simulink model "Sim_test"  (R2016b)
settings: Solver=ode23tb  StartTime=0.0  StopTime=ti(end)  MaxStep=1e-3  EnableMultiTasking=on
InitFcn:
  | fp_sp_k = 12e3;
  | fp_sp_d = 1;
  | weights = 70/6;
  | joint_k = 0*180/pi;
  | joint_d = 0*180/pi;
  | fp_uj_dp_k = 500*180/pi;
  | fp_uj_dp_d = 1*180/pi;
  | fp_uj_ie_k = 500*180/pi;
  | fp_uj_ie_d = 1*180/pi;
values from neighbouring files (symbols this model uses):
  N = length(shin_angles_in.signals.values)    [GaitEmu_code.m]    (also in dy1.m; dy2.m; est_joint.m = size( [body1.trans body2.trans], 1 ); impcont.m)
  s = [-atan((t2.*3.379e-4+t3+t4.*t5.*4.401e-2)./(t4.*cos(q2)));-asin(t2.*1.4870979e-5+t3.*4.401e-2-t4.*t5)]    [FK_af.m]    (also in FK_footimp.m = [atan((ree2_1.*t2.*4.401e-2+ree2_2.*t4+ree2_3.*t3+t5.*t7.*4.; FK_gaitEmul.m = [q1+t2.*t4.*4.234e-1+t3.*t5.*1.5e-3-t2.*t6.*t7.*1.5e-3-5.347; ik.m = [x; y; z]; ik_af.m = FK_af(q))
  sta = [-0.5345 0.03779 -0.0866]    [GaitEmu_code.m]    (also in dy1.m; dy2.m; grn_dyn.m; impcont.m)
  Y = -( reshape( body1.trans', [], 1 ) - reshape( body2.trans', [], 1 ) )    [creat_joint.m]    (also in est_joint.m = -( reshape( body1.trans', [3*N 1] ) - reshape( body2.trans',)
undefined symbols (not defined in the file or in its folder): X, Z
libraries: sm_lib x263, nesl_utility x76, simulink x3, dspstat3 x1
(part 1 of 6)
settings Model: Creator=lcasteli  LastModifiedBy=Leslie
settings SolverCC: ZeroCrossControl=DisableAll
settings DataIOCC: OutputTimes=[0:0.01:t(end)]
settings OptimizationCC: LifeSpan=inf
settings DebuggingCC: SFUnexpectedBacktrackingDiag=warning  SFNoUnconditionalDefaultTransitionDiag=warning  SFExecutionAtInitializationDiag=none
settings GRTTargetCC: TargetLangStandard=C89/C90 (ANSI)  GeneratePreprocessorConditionals=Disable all
settings ConfigComp: CovMetricSettings=dw  CovHtmlReporting=on  CovSaveCumulativeToWorkspaceVar=on  CovSaveSingleToWorkspaceVar=on  CovExternalEMLEnable=off

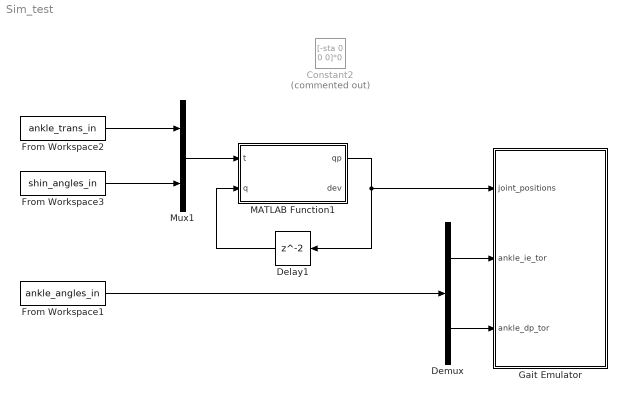
== system Sim_test ==
  Constant2 : Constant  Commented=on  Value=[-sta 0 0 0]*0
  Delay1 : Delay  SampleTime=0.01
  Demux : Demux  Outputs=2
  From Workspace1 : FromWorkspace  VariableName=ankle_angles_in  SampleTime=0
  From Workspace2 : FromWorkspace  VariableName=ankle_trans_in  SampleTime=0
  From Workspace3 : FromWorkspace  VariableName=shin_angles_in  SampleTime=0
  Gait Emulator : Subsystem
  MATLAB Function1 : MATLAB Function  TreatAsAtomicUnit=on
  Mux1 : Mux  Inputs=2
  wires:
  From Workspace1/1 -> Demux/1
  Mux1/1 -> MATLAB Function1/1(t)
  Delay1/1 -> MATLAB Function1/2(q)
  From Workspace2/1 -> Mux1/1
  From Workspace3/1 -> Mux1/2
  MATLAB Function1/1(qp) -> Gait Emulator/1(joint_positions), Delay1/1
  Demux/2 -> Gait Emulator/3(ankle_dp_tor)
  Demux/1 -> Gait Emulator/2(ankle_ie_tor)

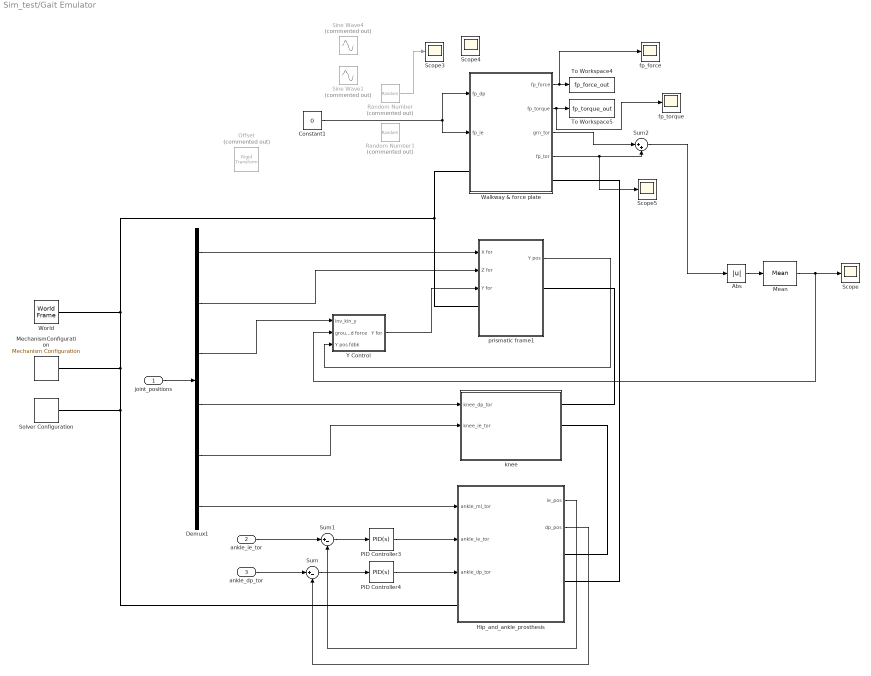
== system Sim_test/Gait Emulator ==
  joint_positions : Inport
  ankle_ie_tor : Inport  Port=2
  ankle_dp_tor : Inport  Port=3
  Abs : Abs
  Constant1 : Constant  Value=0
  Demux1 : Demux  Outputs=6
  Hip_and_ankle_prosthesis : Subsystem
  Mean : dspstat3/Mean  run=off  reset_popup=None  InputProcessing=Columns as channels (frame based)  directionMode=Each column  dimension=1  roiEnable=off  roiType=Rectangles  roiPortion=Entire ROI  roiOutput=Individual statistics for each ROI  roiFlag=off  outputDataTypeStr=Inherit: Same as accumulator  outputLastDataTypeStr=Inherit: Same as accumulator  outputMin=[]  outputMax=[]  roundingMode=Floor  overflowMode=off
  MechanismConfiguration : sm_lib/Utilities/Mechanism Configuration  UniformGravity=Constant  GravityVector=[0 -9.81 0]  GravityUnits=m/s^2  LinearizationDelta=0.001
  Offset : sm_lib/Frames and Transforms/Rigid Transform  Commented=on  TranslationMethod=Cartesian  TranslationStandardOffset=0  TranslationLengthUnit=m  TranslationStandardAxis=+Z  TranslationCartesianOffset=[0.5345 0 -0.03779]  TranslationROffset=0  TranslationROffsetUnits=m  TranslationZOffset=0  TranslationZOffsetUnits=m  TranslationThetaOffset=0  TranslationThetaOffsetUnits=deg  RotationMethod=None  RotationAngleUnits=deg  RotationStandardAxis=+Z  RotationAngle=0.0  RotationArbitraryAxis=[0 0 1]  FollAlignAxisA=+X  BaseAlignAxisA=+Y  FollAlignAxisB=+Y  BaseAlignAxisB=+Z  RotationSequenceAxes=FollowerAxes  RotationSequence=XYX  RotationSequenceAngles=[0 0 0]  RotationSequenceAnglesUnits=deg  RotationMatrix=[1 0 0; 0 1 0; 0 0 1]
  PID Controller3 : simulink/Continuous/PID Controller  Controller=PID  TimeDomain=Continuous-time  SampleTime=-1  IntegratorMethod=Forward Euler  FilterMethod=Forward Euler  Form=Parallel  UseFilter=on  ControllerParametersSource=internal  P=100.231890322584  I=1889.10473464132  D=0.114972413249001  N=105.668461573137  InitialConditionSource=internal  InitialConditionForIntegrator=0  InitialConditionForFilter=0  ExternalReset=none  LimitOutput=off  UpperSaturationLimit=300  LowerSaturationLimit=-300  LinearizeAsGain=on  AntiWindupMode=clamping  Kb=1  TrackingMode=off  Kt=1  PParamMin=[]  PParamMax=[]  IParamMin=[]  IParamMax=[]  DParamMin=[]  DParamMax=[]  NParamMin=[]  NParamMax=[]  KbParamMin=[]  KbParamMax=[]  KtParamMin=[]  KtParamMax=[]  POutMin=[]  POutMax=[]  IOutMin=[]  IOutMax=[]  DOutMin=[]  DOutMax=[]  NOutMin=[]  NOutMax=[]  KbOutMin=[]  KbOutMax=[]  KtOutMin=[]  KtOutMax=[]  IntegratorOutMin=[]  IntegratorOutMax=[]  FilterOutMin=[]  FilterOutMax=[]  SumOutMin=[]  SumOutMax=[]  SumI1OutMin=[]  SumI1OutMax=[]  SumI2OutMin=[]  SumI2OutMax=[]  SumI3OutMin=[]  SumI3OutMax=[]  SumDOutMin=[]  SumDOutMax=[]  SaturationOutMin=[]  SaturationOutMax=[]  IntegratorContinuousStateAttributes=''  IntegratorStateMustResolveToSignalObject=off  IntegratorRTWStateStorageClass=Auto  FilterContinuousStateAttributes=''  FilterStateMustResolveToSignalObject=off  FilterRTWStateStorageClass=Auto  DifferentiatorICPrevScaledInput=0  DifferentiatorOutMin=[]  DifferentiatorOutMax=[]
  PID Controller4 : simulink/Continuous/PID Controller  Controller=PID  TimeDomain=Continuous-time  SampleTime=-1  IntegratorMethod=Forward Euler  FilterMethod=Forward Euler  Form=Parallel  UseFilter=on  ControllerParametersSource=internal  P=98.3049766184944  I=1830.641791322  D=0.171661431514785  N=125.840495387903  InitialConditionSource=internal  InitialConditionForIntegrator=0  InitialConditionForFilter=0  ExternalReset=none  LimitOutput=off  UpperSaturationLimit=300  LowerSaturationLimit=-300  LinearizeAsGain=on  AntiWindupMode=clamping  Kb=1  TrackingMode=off  Kt=1  PParamMin=[]  PParamMax=[]  IParamMin=[]  IParamMax=[]  DParamMin=[]  DParamMax=[]  NParamMin=[]  NParamMax=[]  KbParamMin=[]  KbParamMax=[]  KtParamMin=[]  KtParamMax=[]  POutMin=[]  POutMax=[]  IOutMin=[]  IOutMax=[]  DOutMin=[]  DOutMax=[]  NOutMin=[]  NOutMax=[]  KbOutMin=[]  KbOutMax=[]  KtOutMin=[]  KtOutMax=[]  IntegratorOutMin=[]  IntegratorOutMax=[]  FilterOutMin=[]  FilterOutMax=[]  SumOutMin=[]  SumOutMax=[]  SumI1OutMin=[]  SumI1OutMax=[]  SumI2OutMin=[]  SumI2OutMax=[]  SumI3OutMin=[]  SumI3OutMax=[]  SumDOutMin=[]  SumDOutMax=[]  SaturationOutMin=[]  SaturationOutMax=[]  IntegratorContinuousStateAttributes=''  IntegratorStateMustResolveToSignalObject=off  IntegratorRTWStateStorageClass=Auto  FilterContinuousStateAttributes=''  FilterStateMustResolveToSignalObject=off  FilterRTWStateStorageClass=Auto  DifferentiatorICPrevScaledInput=0  DifferentiatorOutMin=[]  DifferentiatorOutMax=[]
  Random Number : RandomNumber  Commented=on  Variance=1e4  SampleTime=0.1
  Random Number1 : RandomNumber  Commented=on  Variance=4e3  SampleTime=0.1
  Scope{,3..5} (4 alike) : Scope
  Sine Wave1 : Sin  Commented=on  Amplitude=100  Frequency=10  Phase=pi/6  SampleTime=0.001
  Sine Wave4 : Sin  Commented=on  Amplitude=100*2  Frequency=10  SampleTime=0.001
  Solver Configuration : nesl_utility/Solver Configuration  PhysicalDomain=network_engine_domain  SubClassName=solver  LeftPortType=input  RightPortType=generic  Accelerate=off  Tones=[]  Harmonics=[]  SimulateNoise=off  Profile=off  UseLocalSampling=off  EnableSwitchedLinearOptims=on  FrequencyDomain=off  UseCCode=off  RelTol=0.001  AbsTol=1e-06  MinStep=1e-09  ToWorkspace=off  RevertToSquareIcSolve=off  NumHomotopyIterations=100  PhasorMode=off  PhasorModeNumHarmonics=1  OverrideAbsTol=off  DoDC=off  ResidualTolerance=1e-09  UseLocalSolver=off  LocalSolverChoice=NE_BACKWARD_EULER_ADVANCER  LocalSolverSampleTime=0.001  DoFixedCost=off  MaxNonlinIter=3  MaxModeIter=2  LinearAlgebra=Sparse  DelaysMemoryBudget=1024  AutomaticFiltering=on  FilteringTimeConstant=0.001
  Sum : Sum  Inputs=|+-
  Sum1 : Sum  Inputs=|+-
  Sum2 : Sum  Inputs=|++
  To Workspace4 : ToWorkspace  VariableName=fp_force_out  SaveFormat=Structure With Time  SampleTime=-1
  To Workspace5 : ToWorkspace  VariableName=fp_torque_out  SaveFormat=Structure With Time  SampleTime=-1
  Walkway & force plate : Subsystem
  World : sm_lib/Frames and Transforms/World Frame
  Y Control : Subsystem
  fp_force : Scope
  fp_torque : Scope
  "knee " : Subsystem
  prismatic frame1 : Subsystem
  wires:
  joint_positions/1 -> Demux1/1
  Walkway & force plate/2(fp_torque) -> fp_torque/1, To Workspace5/1
  Walkway & force plate/1(fp_force) -> fp_force/1, To Workspace4/1
  Demux1/4 -> "knee "/1(knee_dp_tor)
  Demux1/5 -> "knee "/2(knee_ie_tor)
  Demux1/6 -> Hip_and_ankle_prosthesis/1(ankle_ml_tor)
  Walkway & force plate/3(grn_tor) -> Sum2/1
  Walkway & force plate/4(fp_tor) -> Scope5/1, Sum2/2
  Sum2/1 -> Abs/1
  Abs/1 -> Mean/1
  Mean/1 -> Y Control/2(ground force), Scope/1
  Hip_and_ankle_prosthesis/2(dp_pos) -> Sum/2
  Hip_and_ankle_prosthesis/1(ie_pos) -> Sum1/2
  Sum1/1 -> PID Controller3/1
  Sum/1 -> PID Controller4/1
  Random Number/1 -> Scope3/1
  Constant1/1 -> Walkway & force plate/2(fp_ie), Walkway & force plate/1(fp_dp)
  prismatic frame1/1(Y pos) -> Y Control/3(Y pos fdbk)
  Y Control/1(Y for) -> prismatic frame1/3(Y for)
  Demux1/1 -> prismatic frame1/1(X for)
  Demux1/2 -> prismatic frame1/2(Z for)
  Demux1/3 -> Y Control/1(inv_kin_y)
  PID Controller3/1 -> Hip_and_ankle_prosthesis/2(ankle_ie_tor)
  PID Controller4/1 -> Hip_and_ankle_prosthesis/3(ankle_dp_tor)
  ankle_dp_tor/1 -> Sum/1
  ankle_ie_tor/1 -> Sum1/1
  connections:
  Hip_and_ankle_prosthesis/RConn1 -- "knee "/RConn2
  Walkway & force plate/RConn1 -- Hip_and_ankle_prosthesis/RConn2
  Walkway & force plate/LConn1 -- prismatic frame1/LConn1 -- Hip_and_ankle_prosthesis/LConn1 -- Solver Configuration/RConn1 -- MechanismConfiguration/RConn1 -- World/RConn1
  prismatic frame1/RConn1 -- "knee "/RConn1

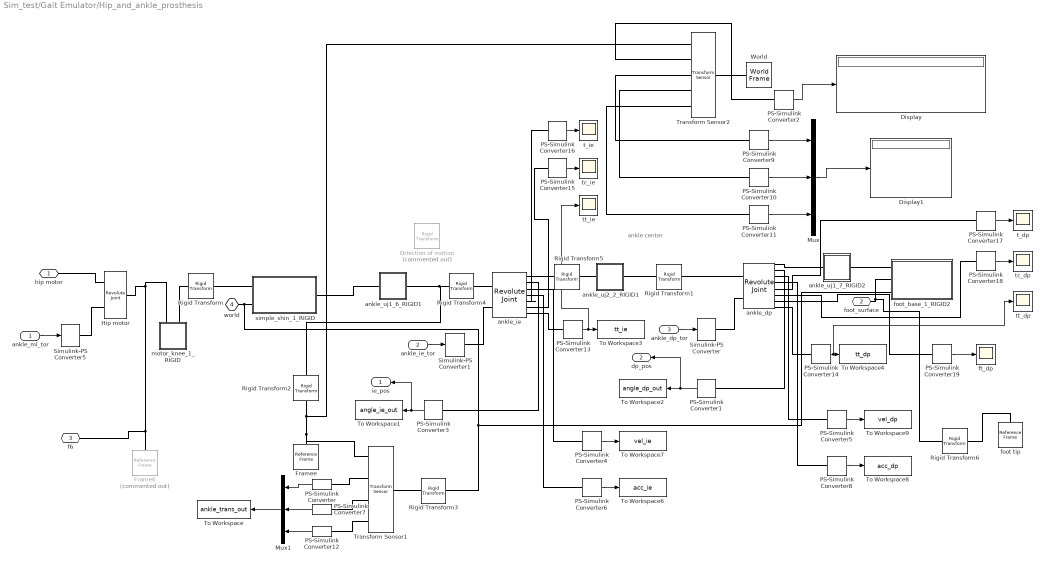
== system Sim_test/Gait Emulator/Hip_and_ankle_prosthesis ==
  note: ankle center
  ankle_ml_tor : Inport
  ankle_ie_tor : Inport  Port=2
  ankle_dp_tor : Inport  Port=3
  Display : Display
  Display1 : Display
  Driection of motion : sm_lib/Frames and Transforms/Rigid Transform  Commented=on  TranslationMethod=None  TranslationStandardOffset=0  TranslationLengthUnit=m  TranslationStandardAxis=+Z  TranslationCartesianOffset=[0 0 0]  TranslationROffset=0  TranslationROffsetUnits=m  TranslationZOffset=0  TranslationZOffsetUnits=m  TranslationThetaOffset=0  TranslationThetaOffsetUnits=deg  RotationMethod=StandardAxis  RotationAngleUnits=deg  RotationStandardAxis=+Z  RotationAngle=0  RotationArbitraryAxis=[0 0 1]  FollAlignAxisA=+X  BaseAlignAxisA=+Y  FollAlignAxisB=+Y  BaseAlignAxisB=+Z  RotationSequenceAxes=FollowerAxes  RotationSequence=XYX  RotationSequenceAngles=[0 0 0]  RotationSequenceAnglesUnits=deg  RotationMatrix=[1 0 0; 0 1 0; 0 0 1]
  Frame6 : sm_lib/Frames and Transforms/Reference Frame  Commented=on
  Framee : sm_lib/Frames and Transforms/Reference Frame
  Hip motor : sm_lib/Joints/Revolute Joint  SenseConstraintForce=off  SenseConstraintForceX=off  SenseConstraintForceY=off  SenseConstraintForceZ=off  SenseConstraintTorque=off  SenseConstraintTorqueX=off  SenseConstraintTorqueY=off  SenseConstraintTorqueZ=off  SenseTotalForce=off  SenseTotalForceX=off  SenseTotalForceY=off  SenseTotalForceZ=off  SenseTotalTorque=off  SenseTotalTorqueX=off  SenseTotalTorqueY=off  SenseTotalTorqueZ=off  CompositeWrenchDir=FollowerOnBase  CompositeWrenchFrame=BaseFrame  EquilibriumPosition=0  EquilibriumPositionUnits=rad  SpringStiffness=joint_k  SpringStiffnessUnits=m*N/rad  DampingCoefficient=joint_d  DampingCoefficientUnits=m*s*N/rad  TorqueActuationMode=ComputedTorque  MotionActuationMode=InputMotion  SensePosition=off  SenseVelocity=off  SenseAcceleration=off  SenseTorqueForce=off  PositionTargetSpecify=off  PositionTargetPriority=Low  PositionTargetValue=0  PositionTargetValueUnits=deg  VelocityTargetSpecify=off  VelocityTargetPriority=High  VelocityTargetValue=0  VelocityTargetValueUnits=deg/s
  Mux : Mux  Inputs=3
  Mux1 : Mux  Inputs=3
  PS-Simulink Converter{,1..19} (20 alike) : nesl_utility/PS-Simulink Converter  PhysicalDomain=network_engine_domain  SubClassName=ps_output  LeftPortType=input  RightPortType=output  PseudoPeriodic=off  Frequencies=[]  Unit=1  AffineConversion=off
  Rigid Transform : sm_lib/Frames and Transforms/Rigid Transform  TranslationMethod=StandardAxis  TranslationStandardOffset=0.15  TranslationLengthUnit=m  TranslationStandardAxis=+Z  TranslationCartesianOffset=[0 0 0]  TranslationROffset=0  TranslationROffsetUnits=m  TranslationZOffset=0  TranslationZOffsetUnits=m  TranslationThetaOffset=0  TranslationThetaOffsetUnits=deg  RotationMethod=StandardAxis  RotationAngleUnits=deg  RotationStandardAxis=+X  RotationAngle=180  RotationArbitraryAxis=[1 0 1]  FollAlignAxisA=+X  BaseAlignAxisA=+Y  FollAlignAxisB=+Y  BaseAlignAxisB=+Z  RotationSequenceAxes=FollowerAxes  RotationSequence=XYX  RotationSequenceAngles=[0 0 0]  RotationSequenceAnglesUnits=deg  RotationMatrix=[1 0 0; 0 1 0; 0 0 1]
  Rigid Transform1 : sm_lib/Frames and Transforms/Rigid Transform  TranslationMethod=None  TranslationStandardOffset=0.15  TranslationLengthUnit=m  TranslationStandardAxis=+Z  TranslationCartesianOffset=[0 0 0]  TranslationROffset=0  TranslationROffsetUnits=m  TranslationZOffset=0  TranslationZOffsetUnits=m  TranslationThetaOffset=0  TranslationThetaOffsetUnits=deg  RotationMethod=StandardAxis  RotationAngleUnits=deg  RotationStandardAxis=+Z  RotationAngle=-90  RotationArbitraryAxis=[1 0 1]  FollAlignAxisA=+X  BaseAlignAxisA=+Y  FollAlignAxisB=+Y  BaseAlignAxisB=+Z  RotationSequenceAxes=FollowerAxes  RotationSequence=XYX  RotationSequenceAngles=[0 0 0]  RotationSequenceAnglesUnits=deg  RotationMatrix=[1 0 0; 0 1 0; 0 0 1]
  Rigid Transform2 : sm_lib/Frames and Transforms/Rigid Transform  TranslationMethod=StandardAxis  TranslationStandardOffset=-8.5e-3  TranslationLengthUnit=m  TranslationStandardAxis=+Z  TranslationCartesianOffset=[0 0 0]  TranslationROffset=0  TranslationROffsetUnits=m  TranslationZOffset=0  TranslationZOffsetUnits=m  TranslationThetaOffset=0  TranslationThetaOffsetUnits=deg  RotationMethod=AlignedAxes  RotationAngleUnits=deg  RotationStandardAxis=+Z  RotationAngle=-90  RotationArbitraryAxis=[1 0 1]  FollAlignAxisA=+X  BaseAlignAxisA=-Z  FollAlignAxisB=+Y  BaseAlignAxisB=-Y  RotationSequenceAxes=FollowerAxes  RotationSequence=XYX  RotationSequenceAngles=[0 0 0]  RotationSequenceAnglesUnits=deg  RotationMatrix=[1 0 0; 0 1 0; 0 0 1]
  Rigid Transform3 : sm_lib/Frames and Transforms/Rigid Transform  TranslationMethod=StandardAxis  TranslationStandardOffset=0.1517  TranslationLengthUnit=m  TranslationStandardAxis=+Y  TranslationCartesianOffset=[0 0 0]  TranslationROffset=0  TranslationROffsetUnits=m  TranslationZOffset=0  TranslationZOffsetUnits=m  TranslationThetaOffset=0  TranslationThetaOffsetUnits=deg  RotationMethod=None  RotationAngleUnits=deg  RotationStandardAxis=+Z  RotationAngle=0.0  RotationArbitraryAxis=[0 0 1]  FollAlignAxisA=+X  BaseAlignAxisA=+Y  FollAlignAxisB=+Y  BaseAlignAxisB=+Z  RotationSequenceAxes=FollowerAxes  RotationSequence=XYX  RotationSequenceAngles=[0 0 0]  RotationSequenceAnglesUnits=deg  RotationMatrix=[1 0 0; 0 1 0; 0 0 1]
  Rigid Transform4 : sm_lib/Frames and Transforms/Rigid Transform  TranslationMethod=StandardAxis  TranslationStandardOffset=-8.5e-3  TranslationLengthUnit=m  TranslationStandardAxis=+Z  TranslationCartesianOffset=[0 0 0]  TranslationROffset=0  TranslationROffsetUnits=m  TranslationZOffset=0  TranslationZOffsetUnits=m  TranslationThetaOffset=0  TranslationThetaOffsetUnits=deg  RotationMethod=None  RotationAngleUnits=deg  RotationStandardAxis=+Z  RotationAngle=0.0  RotationArbitraryAxis=[0 0 1]  FollAlignAxisA=+X  BaseAlignAxisA=+Y  FollAlignAxisB=+Y  BaseAlignAxisB=+Z  RotationSequenceAxes=FollowerAxes  RotationSequence=XYX  RotationSequenceAngles=[0 0 0]  RotationSequenceAnglesUnits=deg  RotationMatrix=[1 0 0; 0 1 0; 0 0 1]
  Rigid Transform5 : sm_lib/Frames and Transforms/Rigid Transform  TranslationMethod=StandardAxis  TranslationStandardOffset=8.5e-3  TranslationLengthUnit=m  TranslationStandardAxis=+Z  TranslationCartesianOffset=[0 0 0]  TranslationROffset=0  TranslationROffsetUnits=m  TranslationZOffset=0  TranslationZOffsetUnits=m  TranslationThetaOffset=0  TranslationThetaOffsetUnits=deg  RotationMethod=None  RotationAngleUnits=deg  RotationStandardAxis=+Z  RotationAngle=0.0  RotationArbitraryAxis=[0 0 1]  FollAlignAxisA=+X  BaseAlignAxisA=+Y  FollAlignAxisB=+Y  BaseAlignAxisB=+Z  RotationSequenceAxes=FollowerAxes  RotationSequence=XYX  RotationSequenceAngles=[0 0 0]  RotationSequenceAnglesUnits=deg  RotationMatrix=[1 0 0; 0 1 0; 0 0 1]
  Rigid Transform6 : sm_lib/Frames and Transforms/Rigid Transform  TranslationMethod=StandardAxis  TranslationStandardOffset=-0.181  TranslationLengthUnit=m  TranslationStandardAxis=+X  TranslationCartesianOffset=[0 0 0]  TranslationROffset=0  TranslationROffsetUnits=m  TranslationZOffset=0  TranslationZOffsetUnits=m  TranslationThetaOffset=0  TranslationThetaOffsetUnits=deg  RotationMethod=None  RotationAngleUnits=deg  RotationStandardAxis=+Z  RotationAngle=0.0  RotationArbitraryAxis=[0 0 1]  FollAlignAxisA=+X  BaseAlignAxisA=+Y  FollAlignAxisB=+Y  BaseAlignAxisB=+Z  RotationSequenceAxes=FollowerAxes  RotationSequence=XYX  RotationSequenceAngles=[0 0 0]  RotationSequenceAnglesUnits=deg  RotationMatrix=[1 0 0; 0 1 0; 0 0 1]
  Simulink-PS Converter : nesl_utility/Simulink-PS Converter  PhysicalDomain=network_engine_domain  SubClassName=ps_input  LeftPortType=input  RightPortType=output  PseudoPeriodic=off  Frequencies=[]  NoiseDistribution=none  NoiseParameters=[]  Unit=1  AffineConversion=off  InputFiltering=on  SimscapeFilterOrder=2  InputFilterTimeConstant=0.001  UdotUserProvided=1
  Simulink-PS Converter1 : nesl_utility/Simulink-PS Converter  PhysicalDomain=network_engine_domain  SubClassName=ps_input  LeftPortType=input  RightPortType=output  PseudoPeriodic=off  Frequencies=[]  NoiseDistribution=none  NoiseParameters=[]  Unit=1  AffineConversion=off  InputFiltering=on  SimscapeFilterOrder=2  InputFilterTimeConstant=0.001  UdotUserProvided=2
  Simulink-PS Converter5 : nesl_utility/Simulink-PS Converter  PhysicalDomain=network_engine_domain  SubClassName=ps_input  LeftPortType=input  RightPortType=output  PseudoPeriodic=off  Frequencies=[]  NoiseDistribution=none  NoiseParameters=[]  Unit=1  AffineConversion=off  InputFiltering=on  SimscapeFilterOrder=2  InputFilterTimeConstant=0.001  UdotUserProvided=2
  To Workspace : ToWorkspace  VariableName=ankle_trans_out  SaveFormat=Structure With Time  SampleTime=-1
  To Workspace1 : ToWorkspace  VariableName=angle_ie_out  SaveFormat=Structure With Time  SampleTime=-1
  To Workspace2 : ToWorkspace  VariableName=angle_dp_out  SaveFormat=Structure With Time  SampleTime=-1
  To Workspace3 : ToWorkspace  VariableName=tt_ie  SaveFormat=Structure With Time  SampleTime=-1
  To Workspace4 : ToWorkspace  VariableName=tt_dp  SaveFormat=Structure With Time  SampleTime=-1
  To Workspace6 : ToWorkspace  VariableName=acc_ie  SaveFormat=Structure With Time  SampleTime=-1
  To Workspace7 : ToWorkspace  VariableName=vel_ie  SaveFormat=Structure With Time  SampleTime=-1
  To Workspace8 : ToWorkspace  VariableName=acc_dp  SaveFormat=Structure With Time  SampleTime=-1
  To Workspace9 : ToWorkspace  VariableName=vel_dp  SaveFormat=Structure With Time  SampleTime=-1
  Transform Sensor1 : sm_lib/Frames and Transforms/Transform Sensor  MeasurementFrame=Base  SenseAngle=off  SenseAxis=off  SenseAngle1=off  SenseAngle2=off  SenseAngle3=off  SenseQ=off  SenseR=off  SenseOmegaX=off  SenseOmegaY=off  SenseOmegaZ=off  SenseOmega1=off  SenseOmega2=off  SenseOmega3=off  SenseQDot=off  SenseRDot=off  SenseAlphaX=off  SenseAlphaY=off  SenseAlphaZ=off  SenseAlpha1=off  SenseAlpha2=off  SenseAlpha3=off  SenseQDDot=off  SenseRDDot=off  SenseX=on  SenseY=on  SenseZ=on  SenseRad=off  SenseAzim=off  SenseDist=off  SenseInc=off  SenseXDot=off  SenseYDot=off  SenseZDot=off  SenseRadDot=off  SenseAzimDot=off  SenseDistDot=off  SenseIncDot=off  SenseXDDot=off  SenseYDDot=off  SenseZDDot=off  SenseRadDDot=off  SenseAzimDDot=off  SenseDistDDot=off  SenseIncDDot=off
  Transform Sensor2 : sm_lib/Frames and Transforms/Transform Sensor  MeasurementFrame=Base  SenseAngle=off  SenseAxis=off  SenseAngle1=off  SenseAngle2=off  SenseAngle3=off  SenseQ=off  SenseR=on  SenseOmegaX=off  SenseOmegaY=off  SenseOmegaZ=off  SenseOmega1=off  SenseOmega2=off  SenseOmega3=off  SenseQDot=off  SenseRDot=off  SenseAlphaX=off  SenseAlphaY=off  SenseAlphaZ=off  SenseAlpha1=off  SenseAlpha2=off  SenseAlpha3=off  SenseQDDot=off  SenseRDDot=off  SenseX=on  SenseY=on  SenseZ=on  SenseRad=off  SenseAzim=off  SenseDist=off  SenseInc=off  SenseXDot=off  SenseYDot=off  SenseZDot=off  SenseRadDot=off  SenseAzimDot=off  SenseDistDot=off  SenseIncDot=off  SenseXDDot=off  SenseYDDot=off  SenseZDDot=off  SenseRadDDot=off  SenseAzimDDot=off  SenseDistDDot=off  SenseIncDDot=off
  World : sm_lib/Frames and Transforms/World Frame
  ankle_dp : sm_lib/Joints/Revolute Joint  SenseConstraintForce=off  SenseConstraintForceX=off  SenseConstraintForceY=off  SenseConstraintForceZ=off  SenseConstraintTorque=on  SenseConstraintTorqueX=off  SenseConstraintTorqueY=off  SenseConstraintTorqueZ=off  SenseTotalForce=on  SenseTotalForceX=off  SenseTotalForceY=off  SenseTotalForceZ=off  SenseTotalTorque=on  SenseTotalTorqueX=off  SenseTotalTorqueY=off  SenseTotalTorqueZ=off  CompositeWrenchDir=FollowerOnBase  CompositeWrenchFrame=BaseFrame  EquilibriumPosition=0  EquilibriumPositionUnits=rad  SpringStiffness=stiff_dp  SpringStiffnessUnits=m*N/rad  DampingCoefficient=damp_dp  DampingCoefficientUnits=m*s*N/rad  TorqueActuationMode=InputTorque  MotionActuationMode=ComputedMotion  SensePosition=on  SenseVelocity=on  SenseAcceleration=on  SenseTorqueForce=on  PositionTargetSpecify=off  PositionTargetPriority=Low  PositionTargetValue=-90  PositionTargetValueUnits=deg  VelocityTargetSpecify=off  VelocityTargetPriority=High  VelocityTargetValue=0  VelocityTargetValueUnits=deg/s
  ankle_ie : sm_lib/Joints/Revolute Joint  SenseConstraintForce=off  SenseConstraintForceX=off  SenseConstraintForceY=off  SenseConstraintForceZ=off  SenseConstraintTorque=on  SenseConstraintTorqueX=off  SenseConstraintTorqueY=off  SenseConstraintTorqueZ=off  SenseTotalForce=off  SenseTotalForceX=off  SenseTotalForceY=off  SenseTotalForceZ=off  SenseTotalTorque=on  SenseTotalTorqueX=off  SenseTotalTorqueY=off  SenseTotalTorqueZ=off  CompositeWrenchDir=FollowerOnBase  CompositeWrenchFrame=BaseFrame  EquilibriumPosition=0  EquilibriumPositionUnits=rad  SpringStiffness=stiff_ie  SpringStiffnessUnits=N*m/rad  DampingCoefficient=damp_ie  DampingCoefficientUnits=m*s*N/rad  TorqueActuationMode=InputTorque  MotionActuationMode=ComputedMotion  SensePosition=on  SenseVelocity=on  SenseAcceleration=on  SenseTorqueForce=on  PositionTargetSpecify=off  PositionTargetPriority=Low  PositionTargetValue=0  PositionTargetValueUnits=deg  VelocityTargetSpecify=off  VelocityTargetPriority=High  VelocityTargetValue=0  VelocityTargetValueUnits=deg/s
  ankle_uj1_6_RIGID1 : Subsystem
  ankle_uj1_7_RIGID2 : Subsystem
  ankle_uj2_2_RIGID1 : Subsystem
  foot tip : sm_lib/Frames and Transforms/Reference Frame
  foot_base_1_RIGID2 : Subsystem
  ft_dp : Scope
  motor_knee_1_RIGID : Subsystem
  simple_shin_1_RIGID : Subsystem
  t_dp : Scope
  t_ie : Scope
  tc_dp : Scope
  tc_ie : Scope
  tt_dp : Scope
  tt_ie : Scope
  hip motor : PMIOPort  Port=1  Side=Right
  foot_surface : PMIOPort  Port=2  Side=Right
  f6 : PMIOPort  Port=3  Side=Right
  world : PMIOPort  Port=4  Side=Left
  ie_pos : Outport
  dp_pos : Outport  Port=2
  wires:
  PS-Simulink Converter1/1 -> dp_pos/1, To Workspace2/1
  PS-Simulink Converter4/1 -> To Workspace7/1
  PS-Simulink Converter5/1 -> To Workspace9/1
  PS-Simulink Converter6/1 -> To Workspace6/1
  PS-Simulink Converter8/1 -> To Workspace8/1
  PS-Simulink Converter9/1 -> Mux/1
  PS-Simulink Converter10/1 -> Mux/2
  PS-Simulink Converter11/1 -> Mux/3
  Mux/1 -> Display1/1
  ankle_ml_tor/1 -> Simulink-PS Converter5/1
  PS-Simulink Converter2/1 -> Display/1
  PS-Simulink Converter3/1 -> ie_pos/1, To Workspace1/1
  ankle_dp_tor/1 -> Simulink-PS Converter/1
  PS-Simulink Converter/1 -> Mux1/1
  PS-Simulink Converter7/1 -> Mux1/2
  PS-Simulink Converter12/1 -> Mux1/3
  Mux1/1 -> To Workspace/1
  PS-Simulink Converter13/1 -> tt_ie/1, To Workspace3/1
  PS-Simulink Converter14/1 -> tt_dp/1, To Workspace4/1
  PS-Simulink Converter18/1 -> tc_dp/1
  PS-Simulink Converter17/1 -> t_dp/1
  PS-Simulink Converter15/1 -> tc_ie/1
  PS-Simulink Converter16/1 -> t_ie/1
  ankle_ie_tor/1 -> Simulink-PS Converter1/1
  PS-Simulink Converter19/1 -> ft_dp/1
  connections:
  ankle_uj2_2_RIGID1/LConn1 -- Rigid Transform5/RConn1
  Rigid Transform1/RConn1 -- ankle_dp/LConn1
  simple_shin_1_RIGID/LConn1 -- Rigid Transform/RConn1
  Rigid Transform/LConn1 -- motor_knee_1_RIGID/RConn2
  ankle_uj2_2_RIGID1/RConn1 -- Rigid Transform1/LConn1
  Hip motor/RConn1 -- motor_knee_1_RIGID/RConn1 -- Frame6/RConn1 -- f6/RConn1
  Hip motor/LConn1 -- hip motor/RConn1
  PS-Simulink Converter4/LConn1 -- ankle_ie/RConn3
  PS-Simulink Converter5/LConn1 -- ankle_dp/RConn3
  PS-Simulink Converter6/LConn1 -- ankle_ie/RConn4
  PS-Simulink Converter8/LConn1 -- ankle_dp/RConn4
  foot_base_1_RIGID2/LConn1 -- ankle_uj1_7_RIGID2/RConn1
  ankle_uj1_7_RIGID2/LConn1 -- ankle_dp/RConn1
  foot_base_1_RIGID2/LConn2 -- Rigid Transform6/LConn1 -- foot_surface/RConn1
  PS-Simulink Converter3/LConn1 -- ankle_ie/RConn2
  PS-Simulink Converter1/LConn1 -- ankle_dp/RConn2
  Transform Sensor2/LConn1 -- World/RConn1
  Transform Sensor2/RConn2 -- PS-Simulink Converter2/LConn1
  Transform Sensor2/RConn3 -- PS-Simulink Converter9/LConn1
  Transform Sensor2/RConn4 -- PS-Simulink Converter10/LConn1
  Transform Sensor2/RConn5 -- PS-Simulink Converter11/LConn1
  Framee/RConn1 -- Rigid Transform2/RConn1 -- Transform Sensor2/RConn1 -- Transform Sensor1/RConn1
  simple_shin_1_RIGID/RConn1 -- ankle_uj1_6_RIGID1/LConn1
  Rigid Transform3/RConn1 -- Transform Sensor1/LConn1
  Transform Sensor1/RConn2 -- PS-Simulink Converter/LConn1
  Transform Sensor1/RConn3 -- PS-Simulink Converter7/LConn1
  Transform Sensor1/RConn4 -- PS-Simulink Converter12/LConn1
  ankle_ie/RConn6 -- PS-Simulink Converter15/LConn1
  ankle_ie/RConn7 -- PS-Simulink Converter13/LConn1
  ankle_ie/RConn5 -- PS-Simulink Converter16/LConn1
  ankle_dp/RConn5 -- PS-Simulink Converter17/LConn1
  ankle_dp/RConn6 -- PS-Simulink Converter18/LConn1
  Rigid Transform2/LConn1 -- ankle_uj1_6_RIGID1/RConn1 -- Rigid Transform4/LConn1
  Rigid Transform4/RConn1 -- ankle_ie/LConn1
  Rigid Transform5/LConn1 -- ankle_ie/RConn1
  ankle_dp/LConn2 -- Simulink-PS Converter/RConn1
  world/RConn1 -- Rigid Transform3/LConn1 -- foot_base_1_RIGID2/LConn3 -- simple_shin_1_RIGID/LConn2
  Simulink-PS Converter5/RConn1 -- Hip motor/LConn2
  ankle_ie/LConn2 -- Simulink-PS Converter1/RConn1
  PS-Simulink Converter14/LConn1 -- ankle_dp/RConn8
  PS-Simulink Converter19/LConn1 -- ankle_dp/RConn7
  Rigid Transform6/RConn1 -- foot tip/RConn1

== system Sim_test/Gait Emulator/Walkway & force plate ==
  fp_dp : Inport
  fp_ie : Inport  Port=2
  FP Contact : Subsystem
  Force Plate : Subsystem
  Ground Contact : Subsystem
  Simulink-PS Converter3 : nesl_utility/Simulink-PS Converter  PhysicalDomain=network_engine_domain  SubClassName=ps_input  LeftPortType=input  RightPortType=output  PseudoPeriodic=off  Frequencies=[]  NoiseDistribution=none  NoiseParameters=[]  Unit=1  AffineConversion=off  InputFiltering=on  SimscapeFilterOrder=2  InputFilterTimeConstant=0.001  UdotUserProvided=1
  Simulink-PS Converter7 : nesl_utility/Simulink-PS Converter  PhysicalDomain=network_engine_domain  SubClassName=ps_input  LeftPortType=input  RightPortType=output  PseudoPeriodic=off  Frequencies=[]  NoiseDistribution=none  NoiseParameters=[]  Unit=1  AffineConversion=off  InputFiltering=on  SimscapeFilterOrder=2  InputFilterTimeConstant=0.0001  UdotUserProvided=1
  Transform2 : sm_lib/Frames and Transforms/Rigid Transform  TranslationMethod=StandardAxis  TranslationStandardOffset=0.1517  TranslationLengthUnit=m  TranslationStandardAxis=+Y  TranslationCartesianOffset=[0 0 0]  TranslationROffset=0  TranslationROffsetUnits=m  TranslationZOffset=0  TranslationZOffsetUnits=m  TranslationThetaOffset=0  TranslationThetaOffsetUnits=deg  RotationMethod=StandardAxis  RotationAngleUnits=deg  RotationStandardAxis=+X  RotationAngle=-90  RotationArbitraryAxis=[0 0 1]  FollAlignAxisA=+X  BaseAlignAxisA=+Y  FollAlignAxisB=+Y  BaseAlignAxisB=+Z  RotationSequenceAxes=FollowerAxes  RotationSequence=XYX  RotationSequenceAngles=[0 0 0]  RotationSequenceAnglesUnits=deg  RotationMatrix=[1 0 0; 0 1 0; 0 0 1]
  walkway_1_RIGID : Subsystem
  world : PMIOPort  Port=1  Side=Left
  foot surface : PMIOPort  Port=2  Side=Right
  fp_force : Outport
  fp_torque : Outport  Port=2
  grn_tor : Outport  Port=3
  fp_tor : Outport  Port=4
  wires:
  fp_dp/1 -> Simulink-PS Converter3/1
  fp_ie/1 -> Simulink-PS Converter7/1
  Force Plate/1(fp_force) -> fp_force/1
  Force Plate/2(fp_torque) -> fp_torque/1
  Ground Contact/1(grn_tor) -> grn_tor/1
  FP Contact/1(fp_tor) -> fp_tor/1
  connections:
  Force Plate/RConn1 -- FP Contact/RConn1
  FP Contact/LConn1 -- Ground Contact/LConn1 -- foot surface/RConn1
  Ground Contact/RConn1 -- Transform2/RConn1
  Simulink-PS Converter3/RConn1 -- Force Plate/LConn2
  Force Plate/LConn3 -- Simulink-PS Converter7/RConn1
  Transform2/LConn1 -- walkway_1_RIGID/LConn1 -- Force Plate/LConn1 -- world/RConn1

== system Sim_test/Gait Emulator/Y Control ==
  inv_kin_y : Inport
  ground force : Inport  Port=2
  Y pos fdbk : Inport  Port=3
  Constant : Constant  Value=0
  PID Controller2 : simulink/Continuous/PID Controller  Controller=PID  TimeDomain=Continuous-time  SampleTime=-1  IntegratorMethod=Forward Euler  FilterMethod=Forward Euler  Form=Parallel  UseFilter=on  ControllerParametersSource=internal  P=81311.420853362  I=160476.881141818  D=5207.81218139461  N=8271.05073782612  InitialConditionSource=internal  InitialConditionForIntegrator=0  InitialConditionForFilter=0  ExternalReset=none  LimitOutput=on  UpperSaturationLimit=2*75*9.81  LowerSaturationLimit=-2*75*9.81  LinearizeAsGain=on  AntiWindupMode=clamping  Kb=1  TrackingMode=off  Kt=1  PParamMin=[]  PParamMax=[]  IParamMin=[]  IParamMax=[]  DParamMin=[]  DParamMax=[]  NParamMin=[]  NParamMax=[]  KbParamMin=[]  KbParamMax=[]  KtParamMin=[]  KtParamMax=[]  POutMin=[]  POutMax=[]  IOutMin=[]  IOutMax=[]  DOutMin=[]  DOutMax=[]  NOutMin=[]  NOutMax=[]  KbOutMin=[]  KbOutMax=[]  KtOutMin=[]  KtOutMax=[]  IntegratorOutMin=[]  IntegratorOutMax=[]  FilterOutMin=[]  FilterOutMax=[]  SumOutMin=[]  SumOutMax=[]  SumI1OutMin=[]  SumI1OutMax=[]  SumI2OutMin=[]  SumI2OutMax=[]  SumI3OutMin=[]  SumI3OutMax=[]  SumDOutMin=[]  SumDOutMax=[]  SaturationOutMin=[]  SaturationOutMax=[]  IntegratorContinuousStateAttributes=''  IntegratorStateMustResolveToSignalObject=off  IntegratorRTWStateStorageClass=Auto  FilterContinuousStateAttributes=''  FilterStateMustResolveToSignalObject=off  FilterRTWStateStorageClass=Auto  DifferentiatorICPrevScaledInput=0  DifferentiatorOutMin=[]  DifferentiatorOutMax=[]
  Sum3 : Sum  Inputs=|+-
  Switch1 : Switch  Criteria=u2 > Threshold
  Y for : Outport
  wires:
  Y pos fdbk/1 -> Sum3/2
  Constant/1 -> Switch1/1
  Sum3/1 -> PID Controller2/1
  PID Controller2/1 -> Switch1/3
  inv_kin_y/1 -> Sum3/1
  Switch1/1 -> Y for/1
  ground force/1 -> Switch1/2

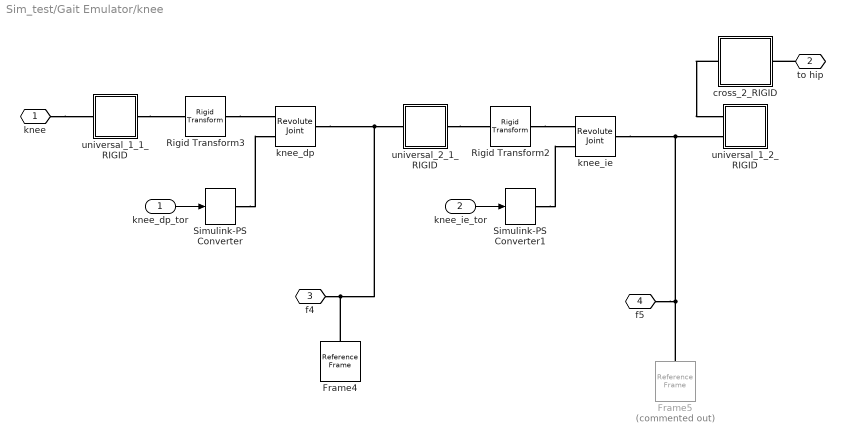
== system Sim_test/Gait Emulator/knee  ==
  knee_dp_tor : Inport
  knee_ie_tor : Inport  Port=2
  Frame4 : sm_lib/Frames and Transforms/Reference Frame
  Frame5 : sm_lib/Frames and Transforms/Reference Frame  Commented=on
  Rigid Transform2 : sm_lib/Frames and Transforms/Rigid Transform  TranslationMethod=None  TranslationStandardOffset=0  TranslationLengthUnit=m  TranslationStandardAxis=+Z  TranslationCartesianOffset=[0 0 0]  TranslationROffset=0  TranslationROffsetUnits=m  TranslationZOffset=0  TranslationZOffsetUnits=m  TranslationThetaOffset=0  TranslationThetaOffsetUnits=deg  RotationMethod=StandardAxis  RotationAngleUnits=deg  RotationStandardAxis=+Z  RotationAngle=-90  RotationArbitraryAxis=[0 0 1]  FollAlignAxisA=+X  BaseAlignAxisA=+Y  FollAlignAxisB=+Y  BaseAlignAxisB=+Z  RotationSequenceAxes=FollowerAxes  RotationSequence=XYX  RotationSequenceAngles=[0 0 0]  RotationSequenceAnglesUnits=deg  RotationMatrix=[1 0 0; 0 1 0; 0 0 1]
  Rigid Transform3 : sm_lib/Frames and Transforms/Rigid Transform  TranslationMethod=StandardAxis  TranslationStandardOffset=-0.034  TranslationLengthUnit=m  TranslationStandardAxis=+Z  TranslationCartesianOffset=[0 0 0]  TranslationROffset=0  TranslationROffsetUnits=m  TranslationZOffset=0  TranslationZOffsetUnits=m  TranslationThetaOffset=0  TranslationThetaOffsetUnits=deg  RotationMethod=StandardAxis  RotationAngleUnits=deg  RotationStandardAxis=+Y  RotationAngle=180  RotationArbitraryAxis=[0 0 1]  FollAlignAxisA=+X  BaseAlignAxisA=+Y  FollAlignAxisB=+Y  BaseAlignAxisB=+Z  RotationSequenceAxes=FollowerAxes  RotationSequence=XYX  RotationSequenceAngles=[0 0 0]  RotationSequenceAnglesUnits=deg  RotationMatrix=[1 0 0; 0 1 0; 0 0 1]
  Simulink-PS Converter : nesl_utility/Simulink-PS Converter  PhysicalDomain=network_engine_domain  SubClassName=ps_input  LeftPortType=input  RightPortType=output  PseudoPeriodic=off  Frequencies=[]  NoiseDistribution=none  NoiseParameters=[]  Unit=1  AffineConversion=off  InputFiltering=on  SimscapeFilterOrder=2  InputFilterTimeConstant=0.001  UdotUserProvided=1
  Simulink-PS Converter1 : nesl_utility/Simulink-PS Converter  PhysicalDomain=network_engine_domain  SubClassName=ps_input  LeftPortType=input  RightPortType=output  PseudoPeriodic=off  Frequencies=[]  NoiseDistribution=none  NoiseParameters=[]  Unit=1  AffineConversion=off  InputFiltering=on  SimscapeFilterOrder=2  InputFilterTimeConstant=0.001  UdotUserProvided=1
  cross_2_RIGID : Subsystem
  knee_dp : sm_lib/Joints/Revolute Joint  SenseConstraintForce=off  SenseConstraintForceX=off  SenseConstraintForceY=off  SenseConstraintForceZ=off  SenseConstraintTorque=off  SenseConstraintTorqueX=off  SenseConstraintTorqueY=off  SenseConstraintTorqueZ=off  SenseTotalForce=off  SenseTotalForceX=off  SenseTotalForceY=off  SenseTotalForceZ=off  SenseTotalTorque=off  SenseTotalTorqueX=off  SenseTotalTorqueY=off  SenseTotalTorqueZ=off  CompositeWrenchDir=FollowerOnBase  CompositeWrenchFrame=BaseFrame  EquilibriumPosition=0  EquilibriumPositionUnits=rad  SpringStiffness=joint_k  SpringStiffnessUnits=m*N/rad  DampingCoefficient=joint_d  DampingCoefficientUnits=m*s*N/rad  TorqueActuationMode=ComputedTorque  MotionActuationMode=InputMotion  SensePosition=off  SenseVelocity=off  SenseAcceleration=off  SenseTorqueForce=off  PositionTargetSpecify=off  PositionTargetPriority=Low  PositionTargetValue=179.9999999999999999  PositionTargetValueUnits=deg  VelocityTargetSpecify=off  VelocityTargetPriority=High  VelocityTargetValue=0  VelocityTargetValueUnits=deg/s
  knee_ie : sm_lib/Joints/Revolute Joint  SenseConstraintForce=off  SenseConstraintForceX=off  SenseConstraintForceY=off  SenseConstraintForceZ=off  SenseConstraintTorque=off  SenseConstraintTorqueX=off  SenseConstraintTorqueY=off  SenseConstraintTorqueZ=off  SenseTotalForce=off  SenseTotalForceX=off  SenseTotalForceY=off  SenseTotalForceZ=off  SenseTotalTorque=off  SenseTotalTorqueX=off  SenseTotalTorqueY=off  SenseTotalTorqueZ=off  CompositeWrenchDir=FollowerOnBase  CompositeWrenchFrame=BaseFrame  EquilibriumPosition=0  EquilibriumPositionUnits=rad  SpringStiffness=joint_k  SpringStiffnessUnits=m*N/rad  DampingCoefficient=joint_d  DampingCoefficientUnits=m*s*N/rad  TorqueActuationMode=ComputedTorque  MotionActuationMode=InputMotion  SensePosition=off  SenseVelocity=off  SenseAcceleration=off  SenseTorqueForce=off  PositionTargetSpecify=off  PositionTargetPriority=Low  PositionTargetValue=90  PositionTargetValueUnits=deg  VelocityTargetSpecify=off  VelocityTargetPriority=High  VelocityTargetValue=0  VelocityTargetValueUnits=deg/s
  universal_1_1_RIGID : Subsystem
  universal_1_2_RIGID : Subsystem
  universal_2_1_RIGID : Subsystem
  knee : PMIOPort  Port=1  Side=Right
  to hip : PMIOPort  Port=2  Side=Right
  f4 : PMIOPort  Port=3  Side=Left
  f5 : PMIOPort  Port=4  Side=Right
  wires:
  knee_dp_tor/1 -> Simulink-PS Converter/1
  knee_ie_tor/1 -> Simulink-PS Converter1/1
  connections:
  universal_1_1_RIGID/RConn1 -- Rigid Transform3/LConn1
  Rigid Transform3/RConn1 -- knee_dp/LConn1
  knee_dp/RConn1 -- f4/RConn1 -- Frame4/RConn1 -- universal_2_1_RIGID/LConn1
  Rigid Transform2/RConn1 -- knee_ie/LConn1
  knee_ie/RConn1 -- Frame5/RConn1 -- f5/RConn1 -- universal_1_2_RIGID/LConn2
  universal_2_1_RIGID/RConn1 -- Rigid Transform2/LConn1
  cross_2_RIGID/LConn1 -- universal_1_2_RIGID/LConn1
  to hip/RConn1 -- cross_2_RIGID/RConn1
  knee/RConn1 -- universal_1_1_RIGID/LConn1
  Simulink-PS Converter1/RConn1 -- knee_ie/LConn2
  Simulink-PS Converter/RConn1 -- knee_dp/LConn2

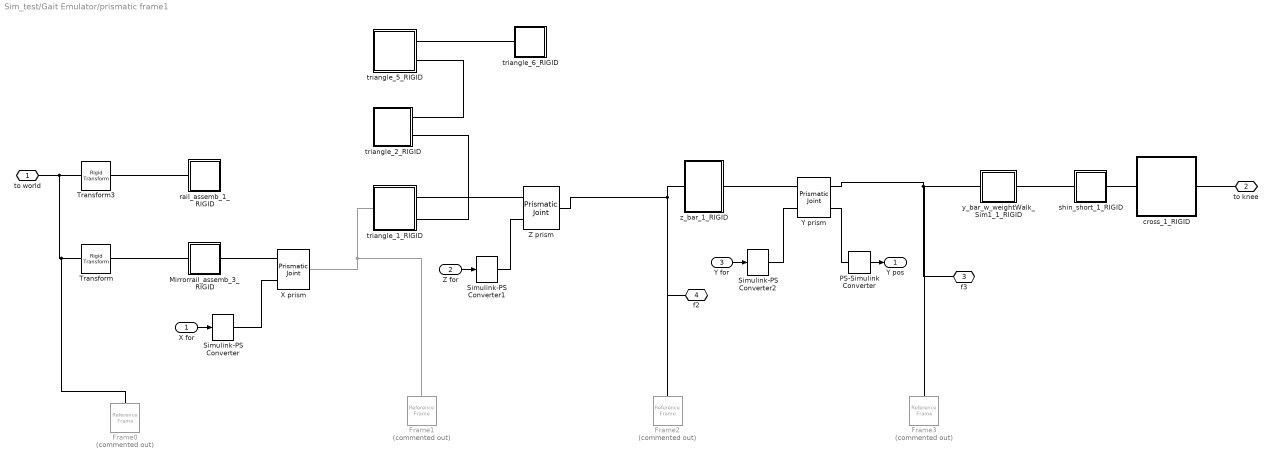
== system Sim_test/Gait Emulator/prismatic frame1 ==
  X for : Inport
  Z for : Inport  Port=2
  Y for : Inport  Port=3
  Frame{0..3} (4 alike) : sm_lib/Frames and Transforms/Reference Frame  Commented=on
  Mirrorrail_assemb_3_RIGID : Subsystem
  PS-Simulink Converter : nesl_utility/PS-Simulink Converter  PhysicalDomain=network_engine_domain  SubClassName=ps_output  LeftPortType=input  RightPortType=output  PseudoPeriodic=off  Frequencies=[]  Unit=1  AffineConversion=off
  Simulink-PS Converter : nesl_utility/Simulink-PS Converter  PhysicalDomain=network_engine_domain  SubClassName=ps_input  LeftPortType=input  RightPortType=output  PseudoPeriodic=off  Frequencies=[]  NoiseDistribution=none  NoiseParameters=[]  Unit=1  AffineConversion=off  InputFiltering=on  SimscapeFilterOrder=2  InputFilterTimeConstant=0.001  UdotUserProvided=1
  Simulink-PS Converter1 : nesl_utility/Simulink-PS Converter  PhysicalDomain=network_engine_domain  SubClassName=ps_input  LeftPortType=input  RightPortType=output  PseudoPeriodic=off  Frequencies=[]  NoiseDistribution=none  NoiseParameters=[]  Unit=1  AffineConversion=off  InputFiltering=on  SimscapeFilterOrder=2  InputFilterTimeConstant=0.001  UdotUserProvided=1
  Simulink-PS Converter2 : nesl_utility/Simulink-PS Converter  PhysicalDomain=network_engine_domain  SubClassName=ps_input  LeftPortType=input  RightPortType=output  PseudoPeriodic=off  Frequencies=[]  NoiseDistribution=none  NoiseParameters=[]  Unit=1  AffineConversion=off  InputFiltering=on  SimscapeFilterOrder=2  InputFilterTimeConstant=0.001  UdotUserProvided=1
  Transform : sm_lib/Frames and Transforms/Rigid Transform  TranslationMethod=Cartesian  TranslationStandardOffset=0  TranslationLengthUnit=m  TranslationStandardAxis=+Z  TranslationCartesianOffset=[3.2000000000000011 1.4389401389271192 0.54097612726828137]  TranslationROffset=0  TranslationROffsetUnits=m  TranslationZOffset=0  TranslationZOffsetUnits=m  TranslationThetaOffset=0  TranslationThetaOffsetUnits=deg  RotationMethod=None  RotationAngleUnits=deg  RotationStandardAxis=+Z  RotationAngle=0.0  RotationArbitraryAxis=[0 0 1]  FollAlignAxisA=+X  BaseAlignAxisA=+Y  FollAlignAxisB=+Y  BaseAlignAxisB=+Z  RotationSequenceAxes=FollowerAxes  RotationSequence=XYX  RotationSequenceAngles=[0 0 0]  RotationSequenceAnglesUnits=deg  RotationMatrix=[1 0 0; 0 1 0; 0 0 1]
  Transform3 : sm_lib/Frames and Transforms/Rigid Transform  TranslationMethod=Cartesian  TranslationStandardOffset=0  TranslationLengthUnit=m  TranslationStandardAxis=+Z  TranslationCartesianOffset=[3.2000000000000011 1.4389401389271192 -0.54097612726828137]  TranslationROffset=0  TranslationROffsetUnits=m  TranslationZOffset=0  TranslationZOffsetUnits=m  TranslationThetaOffset=0  TranslationThetaOffsetUnits=deg  RotationMethod=None  RotationAngleUnits=deg  RotationStandardAxis=+Z  RotationAngle=0.0  RotationArbitraryAxis=[0 0 1]  FollAlignAxisA=+X  BaseAlignAxisA=+Y  FollAlignAxisB=+Y  BaseAlignAxisB=+Z  RotationSequenceAxes=FollowerAxes  RotationSequence=XYX  RotationSequenceAngles=[0 0 0]  RotationSequenceAnglesUnits=deg  RotationMatrix=[1 0 0; 0 1 0; 0 0 1]
  X prism : sm_lib/Joints/Prismatic Joint  SenseConstraintForce=off  SenseConstraintForceX=off  SenseConstraintForceY=off  SenseConstraintForceZ=off  SenseConstraintTorque=off  SenseConstraintTorqueX=off  SenseConstraintTorqueY=off  SenseConstraintTorqueZ=off  SenseTotalForce=off  SenseTotalForceX=off  SenseTotalForceY=off  SenseTotalForceZ=off  SenseTotalTorque=off  SenseTotalTorqueX=off  SenseTotalTorqueY=off  SenseTotalTorqueZ=off  CompositeWrenchDir=FollowerOnBase  CompositeWrenchFrame=BaseFrame  EquilibriumPosition=0  EquilibriumPositionUnits=m  SpringStiffness=joint_k  SpringStiffnessUnits=N/m  DampingCoefficient=joint_d  DampingCoefficientUnits=s*N/m  TorqueActuationMode=ComputedTorque  MotionActuationMode=InputMotion  SensePosition=off  SenseVelocity=off  SenseAcceleration=off  SenseTorqueForce=off  PositionTargetSpecify=off  PositionTargetPriority=Low  PositionTargetValue=-3.2  PositionTargetValueUnits=m  VelocityTargetSpecify=off  VelocityTargetPriority=High  VelocityTargetValue=0  VelocityTargetValueUnits=m/s
  Y prism : sm_lib/Joints/Prismatic Joint  SenseConstraintForce=off  SenseConstraintForceX=off  SenseConstraintForceY=off  SenseConstraintForceZ=off  SenseConstraintTorque=off  SenseConstraintTorqueX=off  SenseConstraintTorqueY=off  SenseConstraintTorqueZ=off  SenseTotalForce=off  SenseTotalForceX=off  SenseTotalForceY=off  SenseTotalForceZ=off  SenseTotalTorque=off  SenseTotalTorqueX=off  SenseTotalTorqueY=off  SenseTotalTorqueZ=off  CompositeWrenchDir=FollowerOnBase  CompositeWrenchFrame=BaseFrame  EquilibriumPosition=0  EquilibriumPositionUnits=m  SpringStiffness=joint_k  SpringStiffnessUnits=N/m  DampingCoefficient=joint_d  DampingCoefficientUnits=s*N/m  TorqueActuationMode=InputTorque  MotionActuationMode=ComputedMotion  SensePosition=on  SenseVelocity=off  SenseAcceleration=off  SenseTorqueForce=off  PositionTargetSpecify=off  PositionTargetPriority=Low  PositionTargetValue=-0.1  PositionTargetValueUnits=m  VelocityTargetSpecify=off  VelocityTargetPriority=High  VelocityTargetValue=0  VelocityTargetValueUnits=m/s
  Z prism : sm_lib/Joints/Prismatic Joint  SenseConstraintForce=off  SenseConstraintForceX=off  SenseConstraintForceY=off  SenseConstraintForceZ=off  SenseConstraintTorque=off  SenseConstraintTorqueX=off  SenseConstraintTorqueY=off  SenseConstraintTorqueZ=off  SenseTotalForce=off  SenseTotalForceX=off  SenseTotalForceY=off  SenseTotalForceZ=off  SenseTotalTorque=off  SenseTotalTorqueX=off  SenseTotalTorqueY=off  SenseTotalTorqueZ=off  CompositeWrenchDir=FollowerOnBase  CompositeWrenchFrame=BaseFrame  EquilibriumPosition=0  EquilibriumPositionUnits=m  SpringStiffness=joint_k  SpringStiffnessUnits=N/m  DampingCoefficient=joint_d  DampingCoefficientUnits=s*N/m  TorqueActuationMode=ComputedTorque  MotionActuationMode=InputMotion  SensePosition=off  SenseVelocity=off  SenseAcceleration=off  SenseTorqueForce=off  PositionTargetSpecify=on  PositionTargetPriority=Low  PositionTargetValue=0  PositionTargetValueUnits=m  VelocityTargetSpecify=off  VelocityTargetPriority=High  VelocityTargetValue=0  VelocityTargetValueUnits=m/s
  cross_1_RIGID : Subsystem
  rail_assemb_1_RIGID : Subsystem
  shin_short_1_RIGID : Subsystem
  triangle_1_RIGID : Subsystem
  triangle_2_RIGID : Subsystem
  triangle_5_RIGID : Subsystem
  triangle_6_RIGID : Subsystem
  y_bar_w_weightWalk_Sim1_1_RIGID : Subsystem
  z_bar_1_RIGID : Subsystem
  to world : PMIOPort  Port=1  Side=Left
  to knee : PMIOPort  Port=2  Side=Right
  f3 : PMIOPort  Port=3  Side=Left
  f2 : PMIOPort  Port=4  Side=Right
  Y pos : Outport
  wires:
  X for/1 -> Simulink-PS Converter/1
  Z for/1 -> Simulink-PS Converter1/1
  Y for/1 -> Simulink-PS Converter2/1
  PS-Simulink Converter/1 -> Y pos/1
  connections:
  cross_1_RIGID/RConn1 -- to knee/RConn1
  to world/RConn1 -- Frame0/RConn1 -- Transform/LConn1 -- Transform3/LConn1
  Frame1/RConn1 -- X prism/RConn1 -- triangle_1_RIGID/LConn1
  Z prism/LConn1 -- triangle_1_RIGID/RConn1
  Mirrorrail_assemb_3_RIGID/RConn1 -- X prism/LConn1
  Y prism/LConn1 -- z_bar_1_RIGID/RConn1
  Z prism/RConn1 -- Frame2/RConn1 -- f2/RConn1 -- z_bar_1_RIGID/LConn1
  Y prism/RConn1 -- Frame3/RConn1 -- f3/RConn1 -- y_bar_w_weightWalk_Sim1_1_RIGID/LConn1
  shin_short_1_RIGID/RConn1 -- cross_1_RIGID/LConn1
  shin_short_1_RIGID/LConn1 -- y_bar_w_weightWalk_Sim1_1_RIGID/RConn1
  triangle_2_RIGID/RConn2 -- triangle_1_RIGID/RConn2
  triangle_6_RIGID/RConn1 -- triangle_5_RIGID/RConn1
  triangle_2_RIGID/RConn1 -- triangle_5_RIGID/RConn2
  Simulink-PS Converter1/RConn1 -- Z prism/LConn2
  Simulink-PS Converter/RConn1 -- X prism/LConn2
  Simulink-PS Converter2/RConn1 -- Y prism/LConn2
  Y prism/RConn2 -- PS-Simulink Converter/LConn1
  Transform3/RConn1 -- rail_assemb_1_RIGID/LConn1
  Transform/RConn1 -- Mirrorrail_assemb_3_RIGID/LConn1

== system Sim_test/Gait Emulator/Hip_and_ankle_prosthesis/ankle_uj1_6_RIGID1 ==
  ReferenceFrame : sm_lib/Frames and Transforms/Reference Frame
  Solid : sm_lib/Body Elements/Solid  InertiaType=Custom  Mass=0.0010110480957103466  MassUnits=kg  CenterOfMass=[-0.023717308914540377 0.015560018734182399 -0.004478891085163238]  CenterOfMassUnits=m  MomentsOfInertia=[7.4638531365509001e-08 6.5681099822924609e-08 3.7045085927626024e-08]  MomentsOfInertiaUnits=kg*m^2  ProductsOfInertia=[0 0 0]  ProductsOfInertiaUnits=kg*m^2  DensityBased=on  Density=1000  DensityUnits=kg/(m^3)  DoExposeReferenceFrame=on  SerializedFrames=<Frames/>  GraphicType=FromGeometry  MarkerShape=Sphere  MarkerSize=10  MarkerSizeUnits=m  GraphicVisPropType=SimpleVisualProperties  GraphicDiffuseColor=[0.792156862745098 0.81960784313725488 0.93333333333333335]  GraphicSpecularColor=[0.5 0.5 0.5 1.0]  GraphicAmbientColor=[0.15 0.15 0.15 1.0]  GraphicEmissiveColor=[0.0 0.0 0.0 1.0]  GraphicShininess=75  GraphicOpacity=1  GeometryShape=FromFile  RectangleSize=[1 1]  RectangleSizeUnits=m  BrickDimensions=[1 1 1]  BrickDimensionUnits=m  CylinderRadius=1  CylinderRadiusUnits=m  CylinderLength=1  CylinderLengthUnits=m  SphereRadius=1  SphereRadiusUnits=m  EllipsoidRadii=[1 1 1]  EllipsoidRadiiUnits=m  ExtrusionCrossSection=[1 1; -1 1; -1 -1; 1 -1]  ExtrusionCrossSectionUnits=m  ExtrusionLength=1  ExtrusionLengthUnits=m  PolygonNumSides=3  PolygonOuterRadius=1  PolygonOuterRadiusUnits=m  ExtGeomFileType=STL  ExtGeomFileName=ankle_uj1_Default_sldprt.STL  ExtGeomFileUnits=m  RevolutionCrossSection=[1 1; 1 -1; 2 -1; 2 1]  RevolutionCrossSectionUnits=m  RevolutionExtent=Full  RevolutionAngle=180  RevolutionAngleUnits=deg
  Transform : sm_lib/Frames and Transforms/Rigid Transform  TranslationMethod=Cartesian  TranslationStandardOffset=0  TranslationLengthUnit=m  TranslationStandardAxis=+Z  TranslationCartesianOffset=[-0.02371730891454241 -0.30761799063290884 -0.0044788910851635243]  TranslationROffset=0  TranslationROffsetUnits=m  TranslationZOffset=0  TranslationZOffsetUnits=m  TranslationThetaOffset=0  TranslationThetaOffsetUnits=deg  RotationMethod=ArbitraryAxis  RotationAngleUnits=rad  RotationStandardAxis=+Z  RotationAngle=2.0943951023931957  RotationArbitraryAxis=[-0.57735026918962573 -0.57735026918962562 -0.57735026918962573]  FollAlignAxisA=+X  BaseAlignAxisA=+Y  FollAlignAxisB=+Y  BaseAlignAxisB=+Z  RotationSequenceAxes=FollowerAxes  RotationSequence=XYX  RotationSequenceAngles=[0 0 0]  RotationSequenceAnglesUnits=deg  RotationMatrix=[1 0 0; 0 1 0; 0 0 1]
  Transform1 : sm_lib/Frames and Transforms/Rigid Transform  TranslationMethod=Cartesian  TranslationStandardOffset=0  TranslationLengthUnit=m  TranslationStandardAxis=+Z  TranslationCartesianOffset=[-0.023717308914540391 0.023780009367091182 0.0040211089148365353]  TranslationROffset=0  TranslationROffsetUnits=m  TranslationZOffset=0  TranslationZOffsetUnits=m  TranslationThetaOffset=0  TranslationThetaOffsetUnits=deg  RotationMethod=ArbitraryAxis  RotationAngleUnits=rad  RotationStandardAxis=+Z  RotationAngle=0  RotationArbitraryAxis=[0 0 0]  FollAlignAxisA=+X  BaseAlignAxisA=+Y  FollAlignAxisB=+Y  BaseAlignAxisB=+Z  RotationSequenceAxes=FollowerAxes  RotationSequence=XYX  RotationSequenceAngles=[0 0 0]  RotationSequenceAnglesUnits=deg  RotationMatrix=[1 0 0; 0 1 0; 0 0 1]
  F : PMIOPort  Port=1  Side=Left
  F1 : PMIOPort  Port=2  Side=Right
  connections:
  ReferenceFrame/RConn1 -- Transform/LConn1 -- Transform1/LConn1 -- Solid/RConn1
  Transform/RConn1 -- F/RConn1
  Transform1/RConn1 -- F1/RConn1
